simulink model "bh_ssc_mech_FINAL"  (R2018a)
settings: Solver=VariableStepAuto  StartTime=0.0  StopTime=3  MaxStep=0.01  RelTol=1e-3  AbsTol=1e-3  EnableMultiTasking=on
undefined symbols (not defined in the file): Mech
libraries: fl_lib x9, nesl_utility x6
CloseFcn:
  | try,close(h1_ssc_solenoid),end
  | clear h1_ssc_solenoid
  | 
  | clear simlog_ssc_solenoid
Description:
  | Solenoid
  | 
  | Copyright 2008-2017 The MathWorks, Inc.
settings Model: Creator=MathWorks  LastModifiedBy=bhorton
settings SolverCC: AutoScaleAbsTol=off
settings DataIOCC: LimitDataPoints=on  SaveFormat=Array
settings OptimizationCC: LifeSpan=inf
settings DebuggingCC: SolverPrmCheckMsg=warning  AllowSymbolicDim=off  SFUnexpectedBacktrackingDiag=warning  SFNoUnconditionalDefaultTransitionDiag=warning  SFExecutionAtInitializationDiag=none
settings HardwareCC: ProdBitPerPointer=32  ProdBitPerSizeT=32  ProdBitPerPtrDiffT=32  ProdLargestAtomicFloat=None  ProdIntDivRoundTo=Undefined  ProdEndianess=Unspecified  ProdWordSize=32  ProdHWDeviceType=32-bit Generic
settings ModelReferenceCC: PropagateSignalLabelsOutOfModel=off
settings CodeAppCC: StateflowObjectComments=on
settings GRTTargetCC: TargetLangStandard=C89/C90 (ANSI)  GeneratePreprocessorConditionals=Disable all
settings ConfigComp: CovMetricSettings=dw  CovHtmlReporting=on  CovSaveCumulativeToWorkspaceVar=on  CovSaveSingleToWorkspaceVar=on  CovExternalEMLEnable=off  CovSFcnEnable=off
settings SimscapeCC: SimscapeLogType=all  SimscapeLogSimulationStatistics=on  SimscapeLogName=simlog_ssc_solenoid  SimscapeLogDataHistory=10000

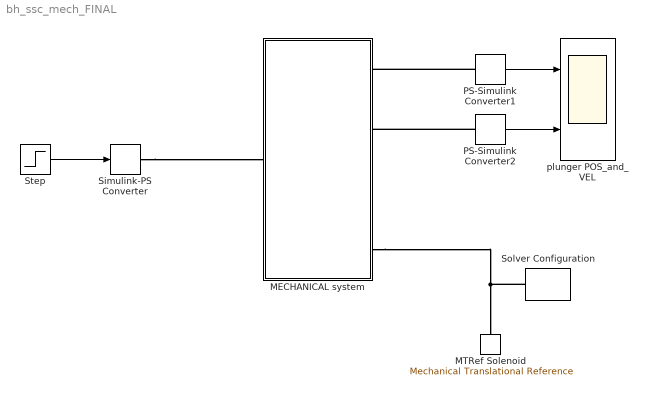
== system bh_ssc_mech_FINAL ==
  MECHANICAL system : Subsystem
  MTRef Solenoid : fl_lib/Mechanical/Translational Elements/Mechanical Translational Reference
  PS-Simulink Converter1 : nesl_utility/PS-Simulink Converter  PhysicalDomain=network_engine_domain  SubClassName=ps_output  LeftPortType=input  RightPortType=output  PseudoPeriodic=off  Frequencies=[]  Unit=m  AffineConversion=off
      settings: AttributesFormatString=units=%<Unit>
  PS-Simulink Converter2 : nesl_utility/PS-Simulink Converter  PhysicalDomain=network_engine_domain  SubClassName=ps_output  LeftPortType=input  RightPortType=output  PseudoPeriodic=off  Frequencies=[]  Unit=m/s  AffineConversion=off
      settings: AttributesFormatString=units=%<Unit>
  Simulink-PS Converter : nesl_utility/Simulink-PS Converter  PhysicalDomain=network_engine_domain  SubClassName=ps_input  LeftPortType=input  RightPortType=output  PseudoPeriodic=off  Frequencies=[]  NoiseDistribution=none  NoiseParameters=[]  Unit=N  AffineConversion=off  FilteringAndDerivatives=provide  SimscapeFilterOrder=1  InputFilterTimeConstant=0.001  UdotUserProvided=0
  Solver Configuration : nesl_utility/Solver Configuration  PhysicalDomain=network_engine_domain  SubClassName=solver  LeftPortType=input  RightPortType=generic  Tones=[]  Harmonics=[]  SimulateNoise=off  Profile=off  UseLocalSampling=off  EnableSwitchedLinearOptims=on  FrequencyDomain=off  UseCCode=off  RelTol=0.001  AbsTol=1e-06  MinStep=1e-09  ToWorkspace=off  RevertToSquareIcSolve=off  NumHomotopyIterations=100  PhasorMode=off  PhasorModeNumHarmonics=1  DoDC=off  ResidualTolerance=1e-09  UseLocalSolver=off  LocalSolverChoice=NE_BACKWARD_EULER_ADVANCER  LocalSolverSampleTime=0.001  DoFixedCost=off  MaxNonlinIter=3  MaxModeIter=2  LinearAlgebra=Sparse  EquationFormulation=NE_TIME_EF  DelaysMemoryBudget=1024  AutomaticFiltering=on  FilteringTimeConstant=0.001
  Step : Step  SampleTime=0
  plunger POS_and_VEL : Scope  NumInputPorts=2
  wires:
  PS-Simulink Converter1/1 -> plunger POS_and_VEL/1
  PS-Simulink Converter2/1 -> plunger POS_and_VEL/2
  Step/1 -> Simulink-PS Converter/1
  connections:
  PS-Simulink Converter1/LConn1 -- MECHANICAL system/RConn1
  PS-Simulink Converter2/LConn1 -- MECHANICAL system/RConn2
  MECHANICAL system/RConn4 -- Solver Configuration/RConn1 -- MTRef Solenoid/LConn1
  Simulink-PS Converter/RConn1 -- MECHANICAL system/LConn1

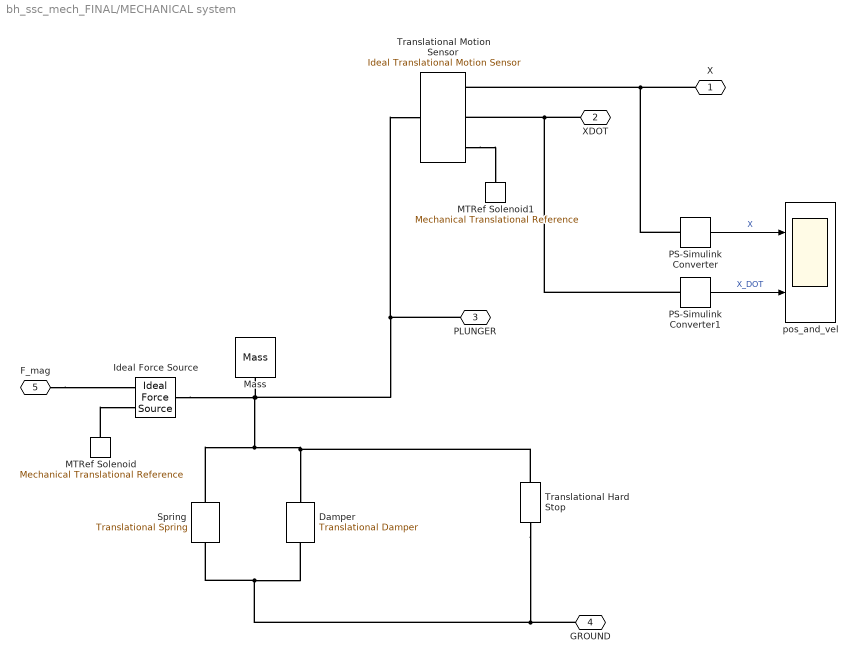
== system bh_ssc_mech_FINAL/MECHANICAL system ==
  Damper : fl_lib/Mechanical/Translational Elements/Translational Damper  D=Mech.C N/(m/s)  v_specify=off  v_priority=High  v=0 m/s  v_nominal_specify=off  v_nominal_unit=m/s  v_nominal_value=1  f_specify=off  f_priority=High  f=0 N  f_nominal_specify=off  f_nominal_unit=N  f_nominal_value=1
  Ideal Force Source : fl_lib/Mechanical/Mechanical Sources/Ideal Force Source
  MTRef Solenoid : fl_lib/Mechanical/Translational Elements/Mechanical Translational Reference
  MTRef Solenoid1 : fl_lib/Mechanical/Translational Elements/Mechanical Translational Reference
  Mass : fl_lib/Mechanical/Translational Elements/Mass  mass=Mech.M kg  v_specify=off  v_priority=High  v=0 m/s  v_nominal_specify=off  v_nominal_unit=m/s  v_nominal_value=1  f_specify=off  f_priority=High  f=0 N  f_nominal_specify=off  f_nominal_unit=N  f_nominal_value=1
  PS-Simulink Converter : nesl_utility/PS-Simulink Converter  PhysicalDomain=network_engine_domain  SubClassName=ps_output  LeftPortType=input  RightPortType=output  PseudoPeriodic=off  Frequencies=[]  Unit=m  AffineConversion=off
      settings: AttributesFormatString=unit=%<Unit>
  PS-Simulink Converter1 : nesl_utility/PS-Simulink Converter  PhysicalDomain=network_engine_domain  SubClassName=ps_output  LeftPortType=input  RightPortType=output  PseudoPeriodic=off  Frequencies=[]  Unit=m/s  AffineConversion=off
      settings: AttributesFormatString=unit=%<Unit>
  Spring : fl_lib/Mechanical/Translational Elements/Translational Spring  spr_rate=Mech.K N/m  v_specify=off  v_priority=High  v=0 m/s  v_nominal_specify=off  v_nominal_unit=m/s  v_nominal_value=1  f_specify=off  f_priority=High  f=0 N  f_nominal_specify=off  f_nominal_unit=N  f_nominal_value=1  x_specify=on  x_priority=High  x=Mech.x_0 m  x_nominal_specify=off  x_nominal_unit=m  x_nominal_value=1
      settings: AttributesFormatString=|
      | DEFLECTION=
      | %<x>
  Translational Motion Sensor : fl_lib/Mechanical/Mechanical Sensors/Ideal Translational Motion Sensor  offset=Mech.x_0 m
      settings: AttributesFormatString=|
      | init_VAL =
      | %<offset> %<offset_unit>
  Translational Hard Stop : fl_lib/Mechanical/Translational Elements/Translational Hard Stop  upper_bnd=Mech.x_max m  lower_bnd=Mech.x_min m  stiff_up=1e6 N/m  stiff_low=1e6 N/m  D_up=500 N/(m/s)  D_low=500 N/(m/s)  model=1  transition=0.1 mm  v_specify=off  v_priority=None  v=0 m/s  v_nominal_specify=off  v_nominal_unit=m/s  v_nominal_value=1  f_specify=off  f_priority=None  f=0 N  f_nominal_specify=off  f_nominal_unit=N  f_nominal_value=1  x_specify=off  x_priority=High  x=0 m  x_nominal_specify=off  x_nominal_unit=m  x_nominal_value=1
      settings: AttributesFormatString=|
      | LOWER_BND = %<lower_bnd>
      | UPPER_BND = %<upper_bnd>
  pos_and_vel : Scope  NumInputPorts=2
  X : PMIOPort  Side=Right
  XDOT : PMIOPort  Port=2  Side=Right
  PLUNGER : PMIOPort  Port=3  Side=Right
  GROUND : PMIOPort  Port=4  Side=Right
  F_mag : PMIOPort  Port=5  Side=Left
  wires:
  PS-Simulink Converter/1 -> pos_and_vel/1  "X"
  PS-Simulink Converter1/1 -> pos_and_vel/2  "X_DOT"
  connections:
  Damper/RConn1 -- Translational Hard Stop/RConn1 -- GROUND/RConn1 -- Spring/RConn1
  F_mag/RConn1 -- Ideal Force Source/RConn1
  MTRef Solenoid/LConn1 -- Ideal Force Source/RConn2
  Translational Motion Sensor/RConn1 -- MTRef Solenoid1/LConn1
  X/RConn1 -- PS-Simulink Converter/LConn1 -- Translational Motion Sensor/RConn3
  XDOT/RConn1 -- PS-Simulink Converter1/LConn1 -- Translational Motion Sensor/RConn2
  PLUNGER/RConn1 -- Translational Motion Sensor/LConn1 -- Translational Hard Stop/LConn1 -- Damper/LConn1 -- Spring/LConn1 -- Ideal Force Source/LConn1 -- Mass/LConn1
